simulink model "udp_receiver"  (R2018b)
settings: Solver=FixedStepAuto  StartTime=0.0  StopTime=inf  FixedStep=0.010  RelTol=1e-3
libraries: dspnetwork x1
settings Model: Creator=nicolai  LastModifiedBy=nicolai

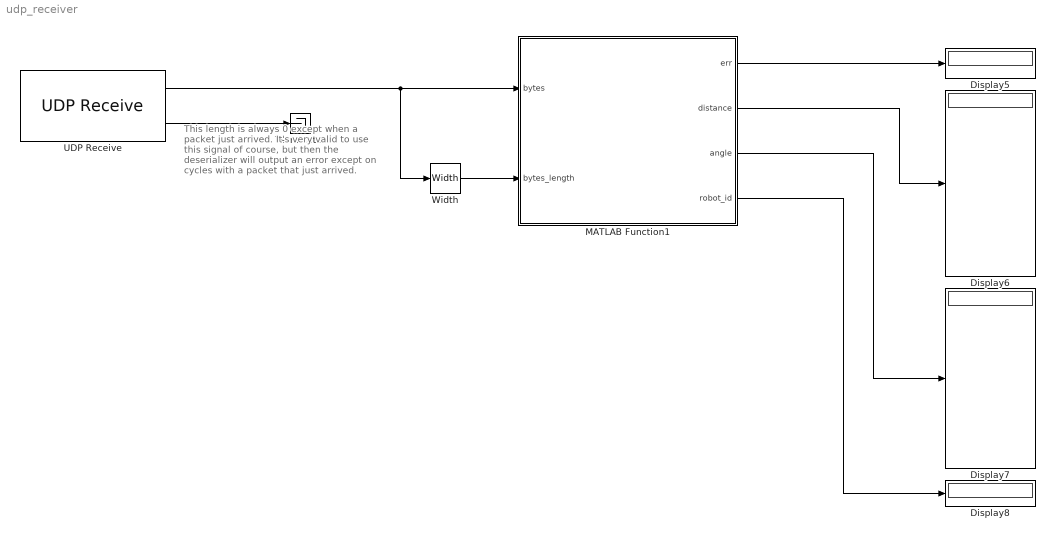
== system udp_receiver ==
  note: This length is always 0 except when a
      | packet just arrived. It's very valid to
      | use this signal of course, but then the
      | deserializer will output an error except
      | on cycles with a packet that just arrived.
  Display{5..8} (4 alike) : Display
  MATLAB Function1 : MATLAB Function  TreatAsAtomicUnit=on
  Terminator : Terminator
  UDP Receive : dspnetwork/UDP Receive  localURL='0.0.0.0'  localPort=25000  remoteURL='0.0.0.0'  remotePort=-1  recvBufferSize=8192  dims=255  signalDatatype=uint8  isVarSize=off  showBlockingTime=off  blockingTime=0  sampletime=1  blockPlatform=[]
      settings: SourceProductName=DSP System Toolbox  SourceProductBaseCode=DS
  Width : Width
  wires:
  UDP Receive/1 -> Width/1, MATLAB Function1/1(bytes)
  Width/1 -> MATLAB Function1/2(bytes_length)
  MATLAB Function1/1(err) -> Display5/1
  MATLAB Function1/2(distance) -> Display6/1
  MATLAB Function1/3(angle) -> Display7/1
  MATLAB Function1/4(robot_id) -> Display8/1
  UDP Receive/2 -> Terminator/1

== matlab function udp_receiver/MATLAB Function1 ==
  data: bytes input; err output; bytes_length input; distance output; angle output; robot_id output
function [err, distance, angle, robot_id] = deserialize_SensorData(bytes, bytes_length)
% deserialize_SensorData Parse microbuf message SensorData (version 1)

err = true;

distance = repmat(single(0), 1, 10);
angle = repmat(single(0), 1, 10);
robot_id = uint8(0);

if bytes_length < 108
    return
end

idx = 1;

[idx, err] = microbuf.check_array(bytes, bytes_length, 21, idx);
if err ;return; end

for i=1:10
    [idx, err, distance(i)] = microbuf.parse_float32(bytes, bytes_length, idx);
    if err ;return; end
end

for i=1:10
    [idx, err, angle(i)] = microbuf.parse_float32(bytes, bytes_length, idx);
    if err ;return; end
end

[idx, err, robot_id] = microbuf.parse_uint8(bytes, bytes_length, idx);
if err ;return; end
[err] = microbuf.check_crc(bytes, bytes_length, idx);

end
